simulink model "Simulador_C2"  (R2018b)
settings: Solver=FixedStepAuto  StartTime=0.0  StopTime=65  FixedStep=Ts3  MaxStep=Ts3  RelTol=1e-3
InitFcn:
  | Ts =0.0200;
  | Ts3= 0.0100;
  | load DatosCrefC2;
StopFcn:
  | clear Ts Ts3 tout;
undefined symbols (not defined in the file or in its folder): sigbuilder_block
settings Model: Creator=jarico  LastModifiedBy=jarico
settings SolverCC: ZeroCrossControl=DisableAll
settings DataIOCC: SaveFormat=StructureWithTime  SignalLogging=off  DSMLogging=off

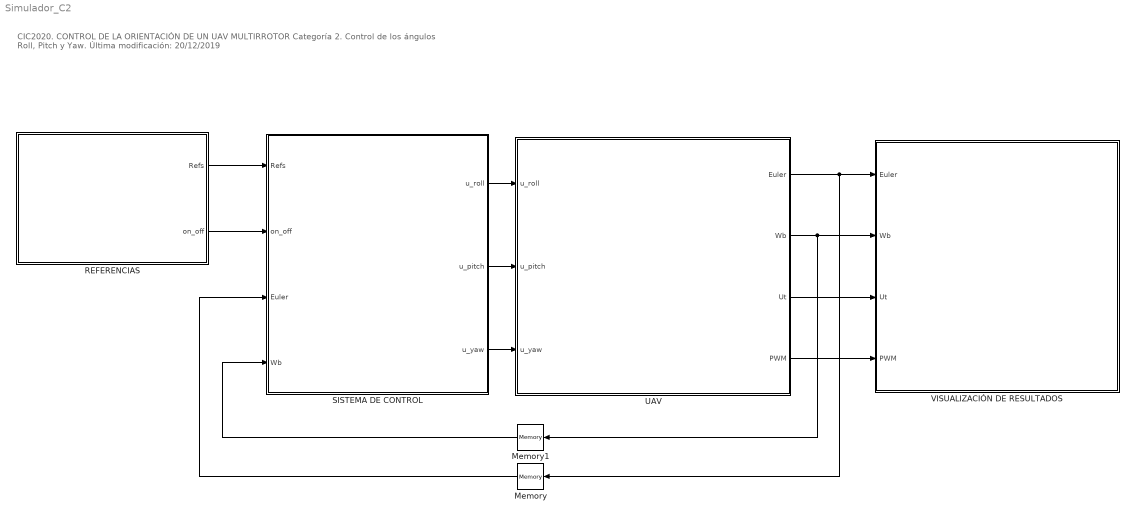
== system Simulador_C2 ==
  note: CIC2020. CONTROL DE LA ORIENTACIÓN DE UN UAV MULTIRROTOR
      |
      | Categoría 2. Control de los ángulos Roll, Pitch y Yaw.
      |
      | Última modificación: 20/12/2019
  Memory : Memory
  Memory1 : Memory
  REFERENCIAS : Subsystem
  SISTEMA DE CONTROL : Subsystem
  UAV : Subsystem  SystemSampleTime=Ts3  mask(Simulador del concurso de Ingeniería de Control CICI2020){v_bat=11, offset=1500, yaw_on=on}
      mask prompts: v_bat "Tensión de la batería"; offset "Offset PID MIX"; yaw_on "Sistema de control de Yaw:"
      mask help:
      | Parámetros configurables del simulador:
      | - Tensión de la batería LiPO de tres celdas. Rango [9, 12.6] voltios.
      | - Offset del algoritmo PID MIX, para simular diferentes cargas útiles soportadas por el UAV. Rango [1000, 2000] micro-segundos.
      | - Sistema de control de ángulo Yaw: Activado (Categoría 2) / Desactivado (Categoría 1)
      mask DialogControl Container7 Prompt: Operación del sistema
      mask Display: image(imread('UAV.png'));
  VISUALIZACIÓN DE RESULTADOS : Subsystem
  wires:
  UAV/4(PWM) -> VISUALIZACIÓN DE RESULTADOS/4(PWM)
  UAV/3(Ut) -> VISUALIZACIÓN DE RESULTADOS/3(Ut)
  UAV/2(Wb) -> VISUALIZACIÓN DE RESULTADOS/2(Wb), Memory1/1
  UAV/1(Euler) -> VISUALIZACIÓN DE RESULTADOS/1(Euler), Memory/1
  SISTEMA DE CONTROL/2(u_pitch) -> UAV/2(u_pitch)
  SISTEMA DE CONTROL/1(u_roll) -> UAV/1(u_roll)
  SISTEMA DE CONTROL/3(u_yaw) -> UAV/3(u_yaw)
  Memory/1 -> SISTEMA DE CONTROL/3(Euler)
  Memory1/1 -> SISTEMA DE CONTROL/4(Wb)
  REFERENCIAS/1(Refs) -> SISTEMA DE CONTROL/1(Refs)
  REFERENCIAS/2(on_off) -> SISTEMA DE CONTROL/2(on_off)

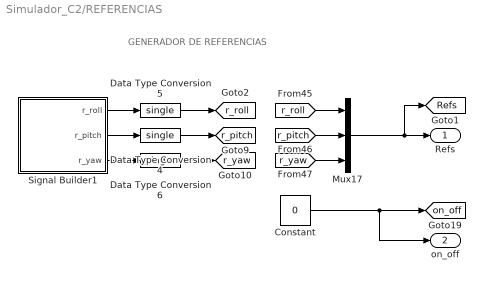
== system Simulador_C2/REFERENCIAS ==
  note: GENERADOR DE REFERENCIAS
  Constant : Constant  Value=0  OutDataTypeStr=int16
  Data Type Conversion4 : DataTypeConversion  OutDataTypeStr=single
  Data Type Conversion5 : DataTypeConversion  OutDataTypeStr=single
  Data Type Conversion6 : DataTypeConversion  OutDataTypeStr=single
  Mux17 : Mux  Inputs=3
  Signal Builder1 : Subsystem  Tag=STV Subsys  LoadFcn=sigbuilder_block('load');  StartFcn=sigbuilder_block('start');  StopFcn=sigbuilder_block('stop');  ClipboardFcn=sigbuilder_block('clipboard');  mask(Sigbuilder block){tuvar=[0:10]}
      mask help: Simulink:masks:SigbuilderBlock_MD
      mask init:
      | if ~strcmp(get_param(bdroot(gcbh),'SimulationStatus'),'stopped') tuvar = sigbuilder_block('maskInit'); end
      settings: CopyFcn=sigbuilder_block('copy');  DeleteFcn=sigbuilder_block('delete');  ModelCloseFcn=sigbuilder_block('modelClose');  PreSaveFcn=sigbuilder_block('preSave');  PauseFcn=sigbuilder_block('pause');  ContinueFcn=sigbuilder_block('continue');  NameChangeFcn=sigbuilder_block('namechange');  OpenFcn=sigbuilder_block('open',[5.4 5.4 1141.2 580.8 ]);  CloseFcn=sigbuilder_block('close');
      mask Display: plot(0, 0, 100, 100,[2, 2, 32, 32, 2], [68, 8, 8, 68, 68],[32, 2], [38, 38], [32, 19, 2],[53, 60, 44], [32, 17, 17, 2],[16, 16, 31, 31]);txt = getActiveGroup(gcbh);text(2, 100, txt,'verticalAlignment', 'top');
  Refs : Outport
  on_off : Outport  Port=2
  tag scope: Refs=global, on_off=global, r_pitch=global, r_roll=global, r_yaw=global
  wires:
  Constant/1 -> on_off/1, [on_off]
  Mux17/1 -> [Refs], Refs/1
  [r_roll] -> Mux17/1
  Data Type Conversion5/1 -> [r_roll]
  Data Type Conversion6/1 -> [r_yaw]
  [r_pitch] -> Mux17/2
  Data Type Conversion4/1 -> [r_pitch]
  [r_yaw] -> Mux17/3
  Signal Builder1/3(r_yaw) -> Data Type Conversion6/1
  Signal Builder1/2(r_pitch) -> Data Type Conversion4/1
  Signal Builder1/1(r_roll) -> Data Type Conversion5/1

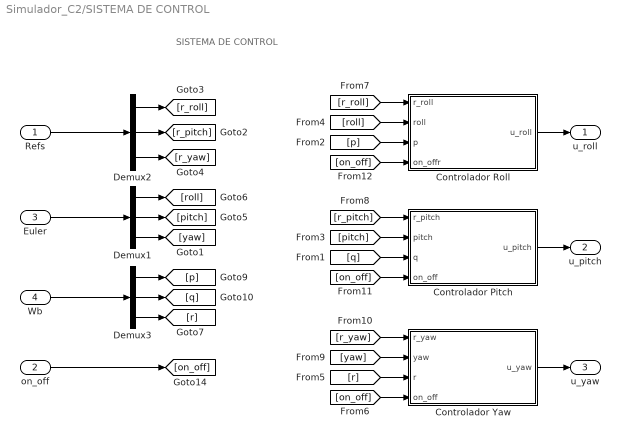
== system Simulador_C2/SISTEMA DE CONTROL ==
  note: SISTEMA DE CONTROL
  Refs : Inport
  on_off : Inport  Port=2
  Euler : Inport  Port=3
  Wb : Inport  Port=4
  Controlador Pitch : Subsystem
  Controlador Roll : Subsystem
  Controlador Yaw : Subsystem
  Demux1 : Demux  Outputs=3
  Demux2 : Demux  Outputs=3
  Demux3 : Demux  Outputs=3
  u_roll : Outport
  u_pitch : Outport  Port=2
  u_yaw : Outport  Port=3
  wires:
  Demux3/1 -> [p]
  Demux3/2 -> [q]
  Demux3/3 -> [r]
  Demux1/1 -> [roll]
  Demux1/2 -> [pitch]
  Demux1/3 -> [yaw]
  [p] -> Controlador Roll/3(p)
  [roll] -> Controlador Roll/2(roll)
  [r_roll] -> Controlador Roll/1(r_roll)
  Refs/1 -> Demux2/1
  Controlador Pitch/1(u_pitch) -> u_pitch/1
  Controlador Roll/1(u_roll) -> u_roll/1
  Demux2/1 -> [r_roll]
  Demux2/2 -> [r_pitch]
  Demux2/3 -> [r_yaw]
  on_off/1 -> [on_off]
  [on_off] -> Controlador Roll/4(on_offr)
  [r_pitch] -> Controlador Pitch/1(r_pitch)
  [pitch] -> Controlador Pitch/2(pitch)
  [q] -> Controlador Pitch/3(q)
  [on_off] -> Controlador Pitch/4(on_off)
  Euler/1 -> Demux1/1
  Wb/1 -> Demux3/1
  Controlador Yaw/1(u_yaw) -> u_yaw/1
  [on_off] -> Controlador Yaw/4(on_off)
  [r] -> Controlador Yaw/3(r)
  [yaw] -> Controlador Yaw/2(yaw)
  [r_yaw] -> Controlador Yaw/1(r_yaw)

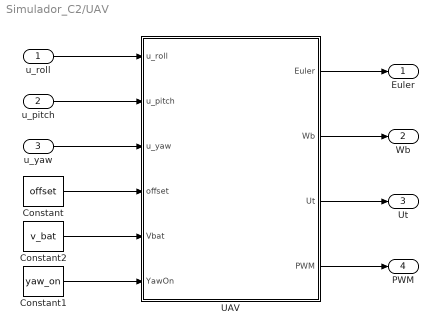
== system Simulador_C2/UAV ==
  u_roll : Inport
  u_pitch : Inport  Port=2
  u_yaw : Inport  Port=3
  Constant : Constant  Value=offset  OutDataTypeStr=int16
  Constant1 : Constant  Value=yaw_on
  Constant2 : Constant  Value=v_bat
  UAV : Subsystem
      mask help: Simulink:masks:GenSFuncDesc_MD
      mask Help: eval('feval(''rtwprivate'',''rtwhelpview'',''rtw_sfcn_block'')');
  Euler : Outport
  Wb : Outport  Port=2
  Ut : Outport  Port=3
  PWM : Outport  Port=4
  wires:
  u_roll/1 -> UAV/1(u_roll)
  u_pitch/1 -> UAV/2(u_pitch)
  u_yaw/1 -> UAV/3(u_yaw)
  Constant/1 -> UAV/4(offset)
  Constant2/1 -> UAV/5(Vbat)
  UAV/3(Ut) -> Ut/1
  UAV/4(PWM) -> PWM/1
  UAV/1(Euler) -> Euler/1
  UAV/2(Wb) -> Wb/1
  Constant1/1 -> UAV/6(YawOn)

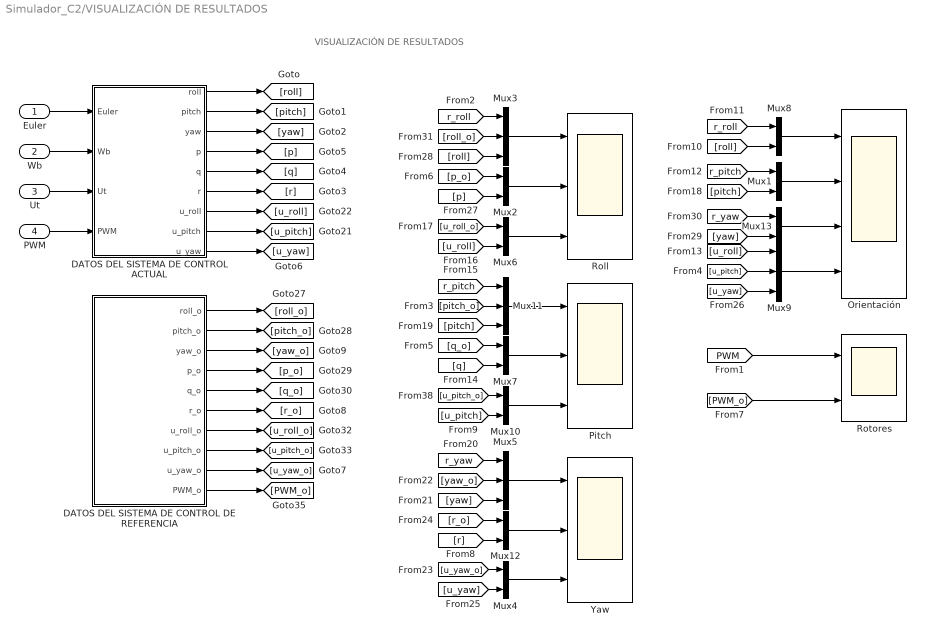
== system Simulador_C2/VISUALIZACIÓN DE RESULTADOS ==
  note: VISUALIZACIÓN DE RESULTADOS
  Euler : Inport
  Wb : Inport  Port=2
  Ut : Inport  Port=3
  PWM : Inport  Port=4
  DATOS DEL SISTEMA DE CONTROL ACTUAL : Subsystem
  DATOS DEL SISTEMA DE CONTROL DE REFERENCIA : Subsystem
  Mux{1..2,4,6..8,10,12..13} (9 alike) : Mux  Inputs=2
  Mux{3,5,9,11} (4 alike) : Mux  Inputs=3
  Orientación : Scope  NumInputPorts=4
  Pitch : Scope  NumInputPorts=3
  Roll : Scope  NumInputPorts=3
  Rotores : Scope  NumInputPorts=2
  Yaw : Scope  NumInputPorts=3
  wires:
  DATOS DEL SISTEMA DE CONTROL DE REFERENCIA/9(u_yaw_o) -> [u_yaw_o]
  DATOS DEL SISTEMA DE CONTROL DE REFERENCIA/6(r_o) -> [r_o]
  DATOS DEL SISTEMA DE CONTROL DE REFERENCIA/3(yaw_o) -> [yaw_o]
  DATOS DEL SISTEMA DE CONTROL ACTUAL/9(u_yaw) -> [u_yaw]
  DATOS DEL SISTEMA DE CONTROL ACTUAL/6(r) -> [r]
  DATOS DEL SISTEMA DE CONTROL ACTUAL/3(yaw) -> [yaw]
  [yaw] -> Mux13/2
  [r_yaw] -> Mux13/1
  Mux13/1 -> Orientación/3
  [u_yaw] -> Mux9/3
  [r_o] -> Mux12/1
  [u_yaw_o] -> Mux4/1
  [yaw] -> Mux5/3
  [yaw_o] -> Mux5/2
  [u_yaw] -> Mux4/2
  [r] -> Mux12/2
  [r_yaw] -> Mux5/1
  Mux4/1 -> Yaw/3
  Mux12/1 -> Yaw/2
  Mux5/1 -> Yaw/1
  Mux11/1 -> Pitch/1
  Mux7/1 -> Pitch/2
  Mux10/1 -> Pitch/3
  [r_pitch] -> Mux11/1
  [q] -> Mux7/2
  [u_pitch] -> Mux10/2
  Mux6/1 -> Roll/3
  Mux2/1 -> Roll/2
  [u_roll] -> Mux6/2
  [p] -> Mux2/2
  PWM/1 -> DATOS DEL SISTEMA DE CONTROL ACTUAL/4(PWM)
  DATOS DEL SISTEMA DE CONTROL ACTUAL/8(u_pitch) -> [u_pitch]
  DATOS DEL SISTEMA DE CONTROL ACTUAL/7(u_roll) -> [u_roll]
  DATOS DEL SISTEMA DE CONTROL ACTUAL/5(q) -> [q]
  DATOS DEL SISTEMA DE CONTROL ACTUAL/4(p) -> [p]
  DATOS DEL SISTEMA DE CONTROL ACTUAL/2(pitch) -> [pitch]
  DATOS DEL SISTEMA DE CONTROL ACTUAL/1(roll) -> [roll]
  Ut/1 -> DATOS DEL SISTEMA DE CONTROL ACTUAL/3(Ut)
  Wb/1 -> DATOS DEL SISTEMA DE CONTROL ACTUAL/2(Wb)
  Euler/1 -> DATOS DEL SISTEMA DE CONTROL ACTUAL/1(Euler)
  DATOS DEL SISTEMA DE CONTROL DE REFERENCIA/4(p_o) -> [p_o]
  DATOS DEL SISTEMA DE CONTROL DE REFERENCIA/5(q_o) -> [q_o]
  DATOS DEL SISTEMA DE CONTROL DE REFERENCIA/10(PWM_o) -> [PWM_o]
  DATOS DEL SISTEMA DE CONTROL DE REFERENCIA/7(u_roll_o) -> [u_roll_o]
  DATOS DEL SISTEMA DE CONTROL DE REFERENCIA/8(u_pitch_o) -> [u_pitch_o]
  DATOS DEL SISTEMA DE CONTROL DE REFERENCIA/1(roll_o) -> [roll_o]
  DATOS DEL SISTEMA DE CONTROL DE REFERENCIA/2(pitch_o) -> [pitch_o]
  [PWM] -> Rotores/1
  [pitch_o] -> Mux11/2
  [pitch] -> Mux11/3
  [r_roll] -> Mux3/1
  Mux9/1 -> Orientación/4
  [u_pitch_o] -> Mux10/1
  [q_o] -> Mux7/1
  [p_o] -> Mux2/1
  [u_roll_o] -> Mux6/1
  Mux3/1 -> Roll/1
  Mux1/1 -> Orientación/2
  [u_pitch] -> Mux9/2
  [u_roll] -> Mux9/1
  [pitch] -> Mux1/2
  [r_pitch] -> Mux1/1
  Mux8/1 -> Orientación/1
  [r_roll] -> Mux8/1
  [roll] -> Mux8/2
  [roll_o] -> Mux3/2
  [roll] -> Mux3/3
  [PWM_o] -> Rotores/2

== system Simulador_C2/REFERENCIAS/Signal Builder1 ==
  Demux : Demux  Tag=STV Demux  Outputs=3
  FromWs : FromWorkspace  Tag=STV FromWs  VariableName=tuvar  SampleTime=0
      SigBuilderData=|
      | common.afterFinalStr = 'Extrapolate'
      | common.sampleTime = 0
      | dataSet.timeRange = [0 65]
      | dataSet.name = 'Group 1'
      | sbobj.Groups.Name = 'Group 1'
      | sbobj.Groups.Signals(1).Name = 'r_roll'
      | sbobj.Groups.Signals(1).XData = [0 5 5 10 10 15 15 20 20 65]
      | sbobj.Groups.Signals(1).YData = [0 0 200 200 0 0 -200 -200 0 0]
      | sbobj.Groups.Signals(2).Name = 'r_pitch'
      | sbobj.Groups.Signals(2).XData = [0 25 25 30 30 35 35 40 40 65]
      | sbobj.Groups.Signals(2).YData = [0 0 200 200 0 0 -200 -200 0.34 0.34]
      | sbobj.Groups.Signals(3).Name = 'r_yaw'
      | sbobj.Groups.Signals(3).XData = [0 45.3 50 55 55 60 65]
      | sbobj.Groups.Signals(3).YData = [0 0 -500 -500 -500 0 0]
      | sbobj.Groups.TimeRange = [0 65]
  r_roll : Outport  Tag=STV Outport
  r_pitch : Outport  Tag=STV Outport  Port=2
  r_yaw : Outport  Tag=STV Outport  Port=3
  wires:
  Demux/1 -> r_roll/1
  FromWs/1 -> Demux/1
  Demux/2 -> r_pitch/1
  Demux/3 -> r_yaw/1

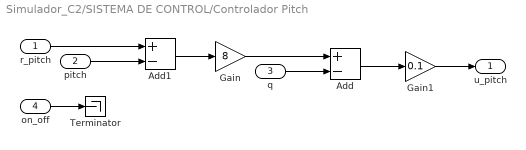
== system Simulador_C2/SISTEMA DE CONTROL/Controlador Pitch ==
  r_pitch : Inport
  pitch : Inport  Port=2
  q : Inport  Port=3
  on_off : Inport  Port=4
  Add : Sum  Inputs=+-
  Add1 : Sum  Inputs=+-
  Gain : Gain  Gain=8
  Gain1 : Gain  Gain=0.1
  Terminator : Terminator
  u_pitch : Outport
  wires:
  Gain1/1 -> u_pitch/1
  Add1/1 -> Gain/1
  on_off/1 -> Terminator/1
  pitch/1 -> Add1/2
  q/1 -> Add/2
  Gain/1 -> Add/1
  Add/1 -> Gain1/1
  r_pitch/1 -> Add1/1

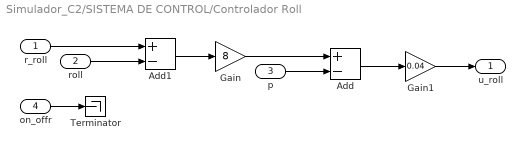
== system Simulador_C2/SISTEMA DE CONTROL/Controlador Roll ==
  r_roll : Inport
  roll : Inport  Port=2
  p : Inport  Port=3
  on_offr : Inport  Port=4
  Add : Sum  Inputs=+-
  Add1 : Sum  Inputs=+-
  Gain : Gain  Gain=8
  Gain1 : Gain  Gain=0.04
  Terminator : Terminator
  u_roll : Outport
  wires:
  r_roll/1 -> Add1/1
  Add/1 -> Gain1/1
  Gain/1 -> Add/1
  p/1 -> Add/2
  roll/1 -> Add1/2
  on_offr/1 -> Terminator/1
  Add1/1 -> Gain/1
  Gain1/1 -> u_roll/1

== system Simulador_C2/SISTEMA DE CONTROL/Controlador Yaw ==
  r_yaw : Inport
  yaw : Inport  Port=2
  r : Inport  Port=3
  on_off : Inport  Port=4
  Add : Sum  Inputs=+-
  Add1 : Sum  Inputs=+-
  Gain : Gain  Gain=8
  Gain1 : Gain  Gain=0.1
  Terminator : Terminator
  u_yaw : Outport
  wires:
  r_yaw/1 -> Add1/1
  Add/1 -> Gain1/1
  Gain/1 -> Add/1
  r/1 -> Add/2
  yaw/1 -> Add1/2
  on_off/1 -> Terminator/1
  Add1/1 -> Gain/1
  Gain1/1 -> u_yaw/1

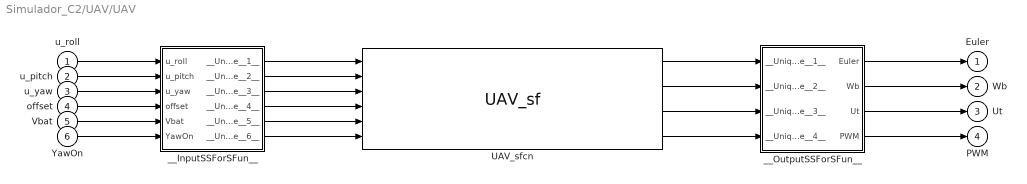
== system Simulador_C2/UAV/UAV ==
  u_roll : Inport
  u_pitch : Inport  Port=2
  u_yaw : Inport  Port=3
  offset : Inport  Port=4
  Vbat : Inport  Port=5
  YawOn : Inport  Port=6
  UAV_sfcn : S-Function  FunctionName=UAV_sf  SFunctionModules=""  SFunctionDeploymentMode=off  EnableBusSupport=off  mask{rtw_sf_name=UAV_sf, showVar=off}
      mask prompts: rtw_sf_name "Simulink:masks:GenSFuncName_MP"; showVar "Simulink:masks:GenSFuncShowModuleList_MP"
      mask help: Simulink:masks:GenSFuncDesc_MD
      mask init:
      | displist = '';
      | if ~strcmp(get_param(gcb, 'FunctionName'), rtw_sf_name);
      |   set_param(gcb, 'FunctionName', rtw_sf_name);
      | end
      | % Check if we are generating code
      | rtw_mode = false;
      | if strcmpi(get_param(bdroot(gcb),'SimulationStatus'),'Initializing')
      | 	rtw_mode = strcmpi(get_param(bdroot(gcb),'BuildingRTWCode'),'on') && ...
      | 		~strcmpi(get_param(bdroot(gcb),'TargetStyle'),'SimulationTarget');
      | end
      | if showVar || rtw_mode
      | 	if exist('rtwsfunc') == 2 | exist('rtwsfunc') == 6
      | 		tmplist = rtwsfunc(rtw_sf_name,gcb);
      | 		tmplist = DAStudio.message('Simulink:masks:GenSFuncListOfModules_IC', tmplist);
      | 	elseif showVar
      | 		tmplist1 = DAStudio.message('Simulink:masks:GenSFuncListOfModules_IC', '');
      |         tmplist2 = DAStudio.message('Simulink:masks:GenSFuncNotLicensed_IC');
      |         tmplist = [tmplist1 tmplist2];
      |  	end
      | end
      | if showVar
      |   displist = tmplist;
      | end
      settings: CopyFcn=|
      | if ~strcmp(get_param(gcb,'Linkstatus'),'none') && ...
      | ~strcmp(get_param(gcb,'Linkstatus'),'implicit')
      |   set_param(gcb,'LinkStatus','none');
      | end
      mask Help: eval('feval(''rtwprivate'',''rtwhelpview'',''rtw_sfcn_block'')');
      mask Display:
      | port_label('input',1,'u_roll');
      | port_label('input',2,'u_pitch');
      | port_label('input',3,'u_yaw');
      | port_label('input',4,'offset');
      | port_label('input',5,'Vbat');
      | port_label('input',6,'YawOn');
      | port_label('output',1,'Euler');
      | port_label('output',2,'Wb');
      | port_label('output',3,'Ut');
      | port_label('output',4,'PWM');
  __InputSSForSFun__ : Subsystem
  __OutputSSForSFun__ : Subsystem
  Euler : Outport
  Wb : Outport  Port=2
  Ut : Outport  Port=3
  PWM : Outport  Port=4
  wires:
  u_roll/1 -> __InputSSForSFun__/1(u_roll)
  u_pitch/1 -> __InputSSForSFun__/2(u_pitch)
  u_yaw/1 -> __InputSSForSFun__/3(u_yaw)
  offset/1 -> __InputSSForSFun__/4(offset)
  Vbat/1 -> __InputSSForSFun__/5(Vbat)
  YawOn/1 -> __InputSSForSFun__/6(YawOn)
  __InputSSForSFun__/1(__UniqueOutportName__1__) -> UAV_sfcn/1
  __InputSSForSFun__/2(__UniqueOutportName__2__) -> UAV_sfcn/2
  __InputSSForSFun__/3(__UniqueOutportName__3__) -> UAV_sfcn/3
  __InputSSForSFun__/4(__UniqueOutportName__4__) -> UAV_sfcn/4
  __InputSSForSFun__/5(__UniqueOutportName__5__) -> UAV_sfcn/5
  __InputSSForSFun__/6(__UniqueOutportName__6__) -> UAV_sfcn/6
  UAV_sfcn/1 -> __OutputSSForSFun__/1(__UniqueInportName__1__)
  UAV_sfcn/2 -> __OutputSSForSFun__/2(__UniqueInportName__2__)
  UAV_sfcn/3 -> __OutputSSForSFun__/3(__UniqueInportName__3__)
  UAV_sfcn/4 -> __OutputSSForSFun__/4(__UniqueInportName__4__)
  __OutputSSForSFun__/1(Euler) -> Euler/1
  __OutputSSForSFun__/2(Wb) -> Wb/1
  __OutputSSForSFun__/3(Ut) -> Ut/1
  __OutputSSForSFun__/4(PWM) -> PWM/1

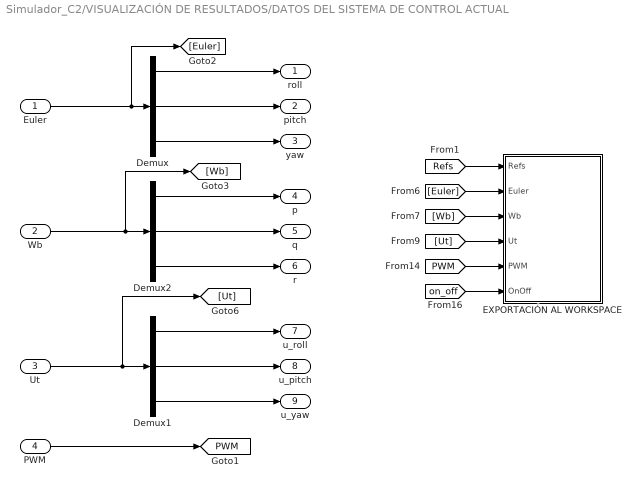
== system Simulador_C2/VISUALIZACIÓN DE RESULTADOS/DATOS DEL SISTEMA DE CONTROL ACTUAL ==
  Euler : Inport
  Wb : Inport  Port=2
  Ut : Inport  Port=3
  PWM : Inport  Port=4
  Demux : Demux  Outputs=3
  Demux1 : Demux  Outputs=3
  Demux2 : Demux  Outputs=3
  EXPORTACIÓN AL WORKSPACE : Subsystem
  roll : Outport
  pitch : Outport  Port=2
  yaw : Outport  Port=3
  p : Outport  Port=4
  q : Outport  Port=5
  r : Outport  Port=6
  u_roll : Outport  Port=7
  u_pitch : Outport  Port=8
  u_yaw : Outport  Port=9
  tag scope: PWM=global
  wires:
  PWM/1 -> [PWM]
  [Euler] -> EXPORTACIÓN AL WORKSPACE/2(Euler)
  [PWM] -> EXPORTACIÓN AL WORKSPACE/5(PWM)
  [Refs] -> EXPORTACIÓN AL WORKSPACE/1(Refs)
  [on_off] -> EXPORTACIÓN AL WORKSPACE/6(OnOff)
  [Ut] -> EXPORTACIÓN AL WORKSPACE/4(Ut)
  [Wb] -> EXPORTACIÓN AL WORKSPACE/3(Wb)
  Demux2/1 -> p/1
  Demux2/2 -> q/1
  Demux1/2 -> u_pitch/1
  Demux/1 -> roll/1
  Demux/3 -> yaw/1
  Euler/1 -> Demux/1, [Euler]
  Demux2/3 -> r/1
  Demux1/1 -> u_roll/1
  Demux1/3 -> u_yaw/1
  Demux/2 -> pitch/1
  Wb/1 -> Demux2/1, [Wb]
  Ut/1 -> [Ut], Demux1/1

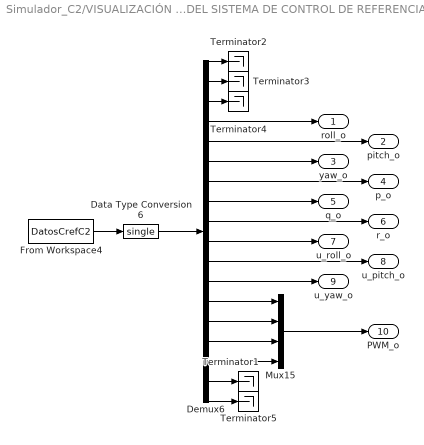
== system Simulador_C2/VISUALIZACIÓN DE RESULTADOS/DATOS DEL SISTEMA DE CONTROL DE REFERENCIA ==
  Data Type Conversion6 : DataTypeConversion  OutDataTypeStr=single
  Demux6 : Demux  Outputs=18
  From Workspace4 : FromWorkspace  VariableName=DatosCrefC2  SampleTime=0
  Mux15 : Mux
  Terminator{1..5} (5 alike) : Terminator
  roll_o : Outport
  pitch_o : Outport  Port=2
  yaw_o : Outport  Port=3
  p_o : Outport  Port=4
  q_o : Outport  Port=5
  r_o : Outport  Port=6
  u_roll_o : Outport  Port=7
  u_pitch_o : Outport  Port=8
  u_yaw_o : Outport  Port=9
  PWM_o : Outport  Port=10
  wires:
  Demux6/18 -> Terminator5/1
  Demux6/17 -> Terminator1/1
  Demux6/12 -> u_yaw_o/1
  Demux6/9 -> r_o/1
  Demux6/11 -> u_pitch_o/1
  Demux6/5 -> pitch_o/1
  Demux6/10 -> u_roll_o/1
  Mux15/1 -> PWM_o/1
  Demux6/7 -> p_o/1
  Demux6/8 -> q_o/1
  Demux6/4 -> roll_o/1
  From Workspace4/1 -> Data Type Conversion6/1
  Demux6/3 -> Terminator4/1
  Demux6/14 -> Mux15/2
  Demux6/16 -> Mux15/4
  Demux6/1 -> Terminator2/1
  Demux6/13 -> Mux15/1
  Data Type Conversion6/1 -> Demux6/1
  Demux6/6 -> yaw_o/1
  Demux6/2 -> Terminator3/1
  Demux6/15 -> Mux15/3

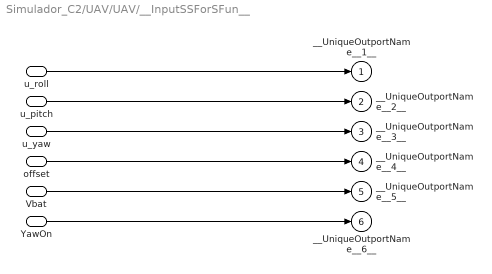
== system Simulador_C2/UAV/UAV/__InputSSForSFun__ ==
  u_roll : Inport
  u_pitch : Inport  Port=2
  u_yaw : Inport  Port=3
  offset : Inport  Port=4
  Vbat : Inport  Port=5
  YawOn : Inport  Port=6
  __UniqueOutportName__1__ : Outport
  __UniqueOutportName__2__ : Outport  Port=2
  __UniqueOutportName__3__ : Outport  Port=3
  __UniqueOutportName__4__ : Outport  Port=4
  __UniqueOutportName__5__ : Outport  Port=5
  __UniqueOutportName__6__ : Outport  Port=6
  wires:
  u_roll/1 -> __UniqueOutportName__1__/1
  u_pitch/1 -> __UniqueOutportName__2__/1
  u_yaw/1 -> __UniqueOutportName__3__/1
  offset/1 -> __UniqueOutportName__4__/1
  Vbat/1 -> __UniqueOutportName__5__/1
  YawOn/1 -> __UniqueOutportName__6__/1

== system Simulador_C2/UAV/UAV/__OutputSSForSFun__ ==
  __UniqueInportName__1__ : Inport
  __UniqueInportName__2__ : Inport  Port=2
  __UniqueInportName__3__ : Inport  Port=3
  __UniqueInportName__4__ : Inport  Port=4
  Euler : Outport
  Wb : Outport  Port=2
  Ut : Outport  Port=3
  PWM : Outport  Port=4
  wires:
  __UniqueInportName__1__/1 -> Euler/1  "euler"
  __UniqueInportName__2__/1 -> Wb/1  "wb"
  __UniqueInportName__3__/1 -> Ut/1
  __UniqueInportName__4__/1 -> PWM/1

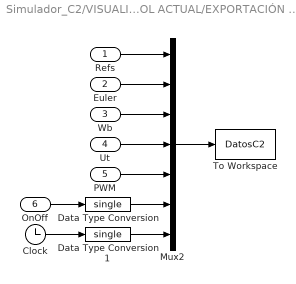
== system Simulador_C2/VISUALIZACIÓN DE RESULTADOS/DATOS DEL SISTEMA DE CONTROL ACTUAL/EXPORTACIÓN AL WORKSPACE ==
  Refs : Inport
  Euler : Inport  Port=2
  Wb : Inport  Port=3
  Ut : Inport  Port=4
  PWM : Inport  Port=5
  OnOff : Inport  Port=6
  Clock : Clock
  Data Type Conversion : DataTypeConversion  OutDataTypeStr=single
  Data Type Conversion1 : DataTypeConversion  OutDataTypeStr=single
  Mux2 : Mux  Inputs=7
  To Workspace : ToWorkspace  VariableName=DatosC2  SaveFormat=Structure With Time  SampleTime=-1
      settings: Decimation=2
  wires:
  PWM/1 -> Mux2/5
  Clock/1 -> Data Type Conversion1/1
  Refs/1 -> Mux2/1
  Mux2/1 -> To Workspace/1
  Data Type Conversion1/1 -> Mux2/7
  Euler/1 -> Mux2/2
  Wb/1 -> Mux2/3
  Data Type Conversion/1 -> Mux2/6
  OnOff/1 -> Data Type Conversion/1
  Ut/1 -> Mux2/4
